simulink model "reference_model_for_fit"  (R2017b)
settings: Solver=FixedStepAuto  StartTime=0.0  StopTime=400  FixedStep=0.1  RelTol=1e-3
InitFcn:
  | % Mass = 10.5;
  | % Lx = 0.19;
  | % Ly = 0.19;
  | % Jz = 0.032;
  | % d = 5e-2;
  | % ua = 0.159;
  | % min_pulse = 0.05;
  | %
  | % % ref model variables
  | % v_pc = 0;
  | % v_sc = 0;
  | % xm0 = -10;
  | % ym0 = 10;
  | % zm0 = 10;
  | % p0 = [xm0 ym0 zm0];
  | % p_dot0 = [0.05, 0.05 -0.05];
  | % angles0 = [30, 30, -30];
  | % w0 = [ 6, -6, 6];
  | % RM.K1 = 2.4e-2 * eye(3);
  | % RM.K2 = 3.6e-3 * eye(3);
  | % K1 = 2.4e-2;
  | % K2 = 3.6e-3;
  | % K3 = diag([0.1, 0.06, 0.096]);
  | % K4= 1e-3*diag([3.7, 1.3, 3.7]);
  | %
StopFcn:
  | % sim_info = stepinfo(Xm_out.Data,Xm_out.Time,0)
undefined symbols (not defined in the file): p0, p_dot0, RM, v_pc
settings Model: Creator=Reza  LastModifiedBy=Reza
settings OptimizationCC: DefaultParameterBehavior=Inlined  UseDivisionForNetSlopeComputation=on  UseFloatMulNetSlope=on  InlineInvariantSignals=on  PassReuseOutputArgsAs=Individual arguments  ZeroExternalMemoryAtStartup=off  ZeroInternalMemoryAtStartup=off  NoFixptDivByZeroProtection=on  EfficientFloat2IntCast=on  LifeSpan=1
settings DebuggingCC: ParameterTunabilityLossMsg=error
settings HardwareCC: ProdLongLongMode=on
settings SFSimCC: MATLABDynamicMemAlloc=off
settings RTWCC: SystemTargetFile=ert.tlc  TemplateMakefile=ert_default_tmf  GenerateReport=on  IncludeHyperlinkInReport=on  LaunchReport=on  TargetLang=C++  GenerateTraceInfo=on  GenerateTraceReport=on  GenerateTraceReportSl=on  GenerateTraceReportSf=on  GenerateTraceReportEml=on
settings CodeAppCC: ForceParamTrailComments=on  IgnoreCustomStorageClasses=off  OperatorAnnotations=on  SimulinkDataObjDesc=on  SFDataObjDesc=on  CustomSymbolStrGlobalVar=rt$N$M  CustomSymbolStrType=$N$M  CustomSymbolStrFcn=$N$M$F  CustomSymbolStrMacro=$N$M  InsertBlockDesc=on
settings ERTTargetCC: TargetLangStandard=C++03 (ISO)  GenerateSampleERTMain=on  IncludeMdlTerminateFcn=off  CombineSignalStateStructs=on  SupportAbsoluteTime=off  MultiInstanceERTCode=on  CodeInterfacePackaging=C++ class  SupportComplex=off  SupportContinuousTime=on  InlinedParameterPlacement=NonHierarchical  RootIOFormat=Structure reference  ERTCustomFileTemplate=example_file_process.tlc  ERTFilePackagingFormat=CompactWithDataFile

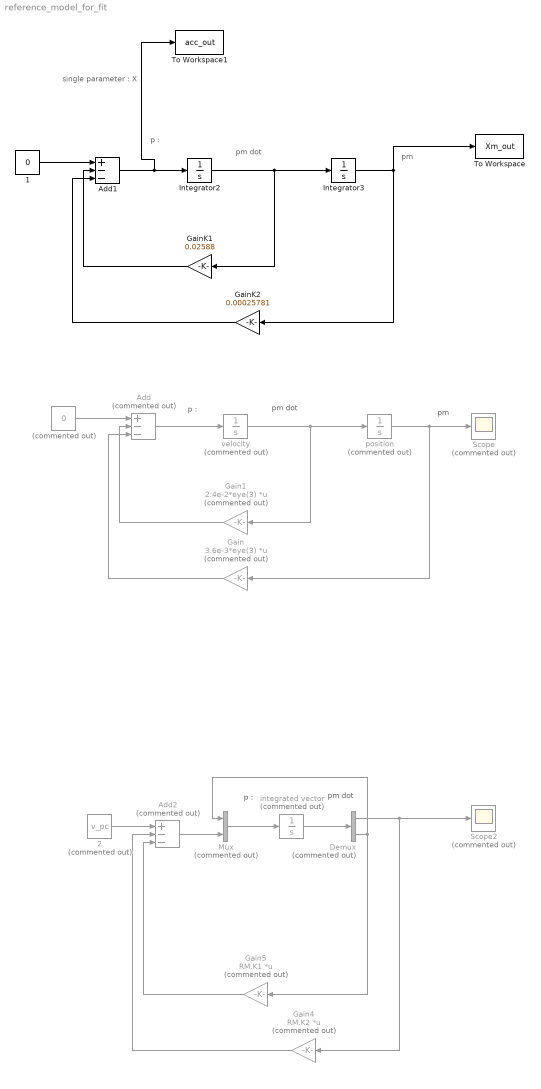
== system reference_model_for_fit ==
  note: single parameter : X
  note: p :
  note: pm
  note: pm dot
  note: p :
  note: pm
  note: pm dot
  note: pm dot
  note: p :
  " " : Constant  Commented=on  Value=0
  " 1" : Constant  Value=0
  " 2" : Constant  Commented=on  Value=v_pc
  Add : Sum  Commented=on  Inputs=+--
  Add1 : Sum  Inputs=+--
  Add2 : Sum  Commented=on  Inputs=+--
  Demux : Demux  Commented=on  Outputs=2
  Gain : Gain  Commented=on  Gain=3.6e-3*eye(3)  Multiplication=Matrix(K*u)
  Gain1 : Gain  Commented=on  Gain=2.4e-2*eye(3)  Multiplication=Matrix(K*u)
  Gain4 : Gain  Commented=on  Gain=RM.K2  Multiplication=Matrix(K*u)
  Gain5 : Gain  Commented=on  Gain=RM.K1  Multiplication=Matrix(K*u)
  GainK1 : Gain  Gain=0.02588
  GainK2 : Gain  Gain=0.00025781
  Integrator2 : Integrator
  Integrator3 : Integrator  InitialCondition=10
  Mux : Mux  Commented=on  Inputs=2
  Scope : Scope  Commented=on
  Scope2 : Scope  Commented=on
  To Workspace : ToWorkspace  VariableName=Xm_out  SaveFormat=Timeseries  SampleTime=-1
  To Workspace1 : ToWorkspace  VariableName=acc_out  SaveFormat=Timeseries  SampleTime=-1
  integrated vector : Integrator  Commented=on  InitialCondition=[p0 p_dot0]
  position : Integrator  Commented=on  InitialCondition=[-10 10 10]
  velocity : Integrator  Commented=on  InitialCondition=[0.05 0.05 -0.05]
  wires:
  position/1 -> Gain/1, Scope/1
  velocity/1 -> Gain1/1, position/1
  Add/1 -> velocity/1
  Gain1/1 -> Add/2
  Gain/1 -> Add/3
  " "/1 -> Add/1
  " 1"/1 -> Add1/1
  GainK2/1 -> Add1/3
  GainK1/1 -> Add1/2
  Integrator2/1 -> Integrator3/1, GainK1/1
  Integrator3/1 -> To Workspace/1, GainK2/1
  " 2"/1 -> Add2/1
  integrated vector/1 -> Demux/1
  Gain5/1 -> Add2/3
  Gain4/1 -> Add2/2
  Demux/1 -> Scope2/1, Gain4/1
  Add2/1 -> Mux/2
  Mux/1 -> integrated vector/1
  Demux/2 -> Gain5/1, Mux/1
  Add1/1 -> To Workspace1/1, Integrator2/1
